simulink model "two_generators_loadFlow"  (R2014a)
settings: Solver=ode23tb  StartTime=0.0  StopTime=10  MaxStep=0.2  RelTol=1e-4
PreLoadFcn:
  | % -- Recommended Settings --
  | %
  | %  Simulink:
  | %      Solver: Ode23tb
  | %      Relative tolerance = 1e-4
  | %      Max step size = 0.2
  | %
  | %  Powergui:
  |          Ts = 0; % (continuous electrical model)
  | %
  | %
  | % ----------------------------------
undefined symbols (not defined in the file): D1, Delta
libraries: powerlib x6
settings Model: Creator=scastro  LastModifiedBy=cosorio
settings DebuggingCC: UnderspecifiedInitializationDetection=Classic  MultiTaskDSMMsg=warning  MultiTaskCondExecSysMsg=none  UnconnectedInputMsg=none  UnconnectedOutputMsg=none  UnconnectedLineMsg=none
settings RTWCC: IncludeERTFirstTime=on

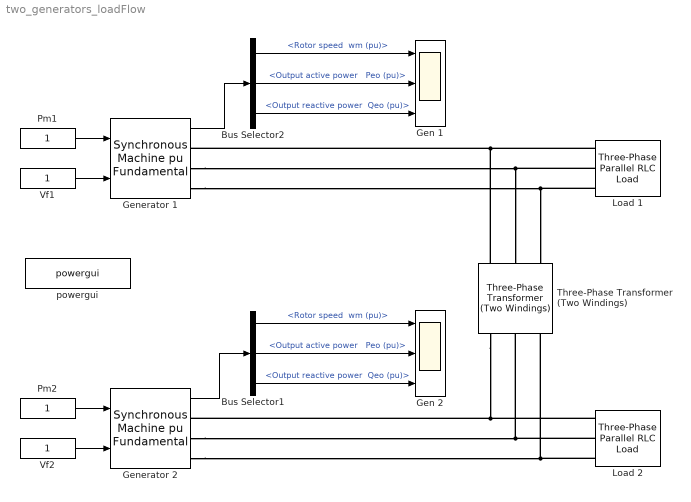
== system two_generators_loadFlow ==
  Bus Selector1 : BusSelector  OutputSignals="Mechanical.Rotor speed  wm (pu),Output active power   Peo (pu),Output reactive power  Qeo (pu)"
  Bus Selector2 : BusSelector  OutputSignals="Mechanical.Rotor speed  wm (pu),Output active power   Peo (pu),Output reactive power  Qeo (pu)"
  Gen 1 : Scope  NumInputPorts=3
      settings: YMin=0~0~0  YMax=2~2~2
  Gen 2 : Scope  NumInputPorts=3
      settings: YMin=0~0~0  YMax=2~2~2  SaveName=ScopeData2
  Generator 1 : powerlib/Machines/Synchronous Machine pu Fundamental  PresetModel=No  MechanicalLoad=Mechanical power Pm  ShowDetailedParameters=on  RotorType=Salient-pole  Units=per unit fundamental parameters  MeasurementBus=off  NominalParameters="[ 50e6  1200   60]"  Stator="[ 2.85E-03  0.114  1.19  0.36 ]"  Field="[ 5.79E-04  0.114]"  Dampers2=[0.0652, 0.5134, 0.0287, 0.2553, 7.765e-3, 0.9167 ]  Dampers1="[ 1.17E-02  0.182  1.97E-02  0.384 ]"  Mechanical=[ 4 0 4]  PolePairs=4  InitialConditions="[ 0  0  0  0  0  0  0  0  1 ]"  SetSaturation=off  Saturation=[0.6404,0.7127,0.8441,0.9214,0.9956,1.082,1.19,1.316,1.457;0.7,0.7698,0.8872,0.9466,0.9969,1.046,1.1,1.151,1.201]  LoadFlowParameters=[4 35000000 1200 0 15000000]  TsPowergui=0  TsBlock=-1  IterativeModel=Trapezoidal non iterative  BusType=swing  Pref=0  Qref=0  Qmin=-inf  Qmax=inf  PLF=0  QLF=0
      settings: AttributesFormatString=%<NominalParameters>
  Generator 2 : powerlib/Machines/Synchronous Machine pu Fundamental  PresetModel=No  MechanicalLoad=Mechanical power Pm  ShowDetailedParameters=on  RotorType=Salient-pole  Units=per unit fundamental parameters  MeasurementBus=off  NominalParameters="[ 50e6  2400   60]"  Stator="[ 2.85E-03  0.114  1.19  0.36 ]"  Field="[ 5.79E-04  0.114]"  Dampers2=[0.0652, 0.5134, 0.0287, 0.2553, 7.765e-3, 0.9167 ]  Dampers1="[ 1.17E-02  0.182  1.97E-02  0.384 ]"  Mechanical=[ 4 0 4]  PolePairs=4  InitialConditions="[ 0  0  0  0  0  0  0  0  1 ]"  SetSaturation=off  Saturation=[0.6404,0.7127,0.8441,0.9214,0.9956,1.082,1.19,1.316,1.457;0.7,0.7698,0.8872,0.9466,0.9969,1.046,1.1,1.151,1.201]  LoadFlowParameters=[2 40000000 1200 0 0]  TsPowergui=0  TsBlock=-1  IterativeModel=Trapezoidal non iterative  BusType=swing  Pref=0  Qref=0  Qmin=-inf  Qmax=inf  PLF=0  QLF=0
      settings: AttributesFormatString=%<NominalParameters>
  Load 1 : powerlib/Elements/Three-Phase Parallel RLC Load  LConnTagsString=A|B|C  Configuration=Y (grounded)  NominalVoltage=1200  NominalFrequency=60  ActivePower=40e6  InductivePower=0  CapacitivePower=0  Measurements=None  LoadType=constant Z
      settings: AttributesFormatString=|
      | P = %<ActivePower> W
      | Q = %<InductivePower> var
  Load 2 : powerlib/Elements/Three-Phase Parallel RLC Load  LConnTagsString=A|B|C  Configuration=Y (grounded)  NominalVoltage=2400  NominalFrequency=60  ActivePower=30e6  InductivePower=25e6  CapacitivePower=0  Measurements=None  LoadType=constant Z
      settings: AttributesFormatString=|
      | P = %<ActivePower> W
      | Q = %<InductivePower> var
  Pm1 : Constant
  Pm2 : Constant
  Three-Phase Transformer (Two Windings) : powerlib/Elements/Three-Phase Transformer (Two Windings)  Winding1Connection=Yg  UNITS=pu  NominalPower=[ 50e6 , 60 ]  Winding1=[ 2400 , 0.002 , 0.08 ]  Winding2Connection=Delta (D1)  Winding2=[ 1200 , 0.002 , 0.08 ]  SetSaturation=off  Rm=500  Lm=500  Saturation=[ 0,0 ; 0.0024,1.2 ; 1.0,1.52 ]  Hysteresis=off  DataFile='hysteresis'  SetInitialFlux=off  InitialFluxes=[ 0.8 , -0.8 , 0.7 ]  Measurements=None  MoreParameters=off  BreakLoop=off  DataType=off  TransfoNumber=1
  Vf1 : Constant
  Vf2 : Constant
  powergui : powerlib/powergui  Priority=1  SimulationMode=Continuous  SolverType=Tustin  SampleTime=1e-4  frequency=60  SPID=off  DisableSnubberDevices=off  DisableRonSwitches=off  DisableVfSwitches=off  SwTol=0  Interpol=off  DisplayEquations=off  Ts=0  methode=off  frequencyindice=60  Pbase=100e6  ErrMax=0.0001  Iterations=50  UnitsV=kV  UnitsW=MW  FunctionMessages=off  echomessages=off  HookPort=off  EnableUseOfTLC=off  x0status=blocks  RestoreLinks=warning  ResistiveCurrentMeasurement=off  Frange=[0:2:500]  Ylog=off  Xlog=on  ShowGrid=off  save=off  variable=ZData  structure=0  ZoomFFT=off  StartTime=0.0  cycles=1  DisplayStyle=1  fundamental=60  FreqAxis=off  MaxFrequency=1000  frequencyindicesteady=1  RmsSteady=1  display=off
  wires:
  Vf1/1 -> Generator 1/2
  Vf2/1 -> Generator 2/2
  Generator 2/1 -> Bus Selector1/1
  Bus Selector1/1 -> Gen 2/1  "<Rotor speed  wm (pu)>"
  Pm1/1 -> Generator 1/1
  Pm2/1 -> Generator 2/1
  Bus Selector1/2 -> Gen 2/2  "<Output active power   Peo (pu)>"
  Bus Selector1/3 -> Gen 2/3  "<Output reactive power  Qeo (pu)>"
  Generator 1/1 -> Bus Selector2/1
  Bus Selector2/1 -> Gen 1/1  "<Rotor speed  wm (pu)>"
  Bus Selector2/2 -> Gen 1/2  "<Output active power   Peo (pu)>"
  Bus Selector2/3 -> Gen 1/3  "<Output reactive power  Qeo (pu)>"
  connections:
  Three-Phase Transformer (Two Windings)/LConn1 -- Load 2/LConn1 -- Generator 2/RConn1
  Generator 1/RConn3 -- Three-Phase Transformer (Two Windings)/RConn3 -- Load 1/LConn3
  Generator 1/RConn2 -- Three-Phase Transformer (Two Windings)/RConn2 -- Load 1/LConn2
  Three-Phase Transformer (Two Windings)/RConn1 -- Load 1/LConn1 -- Generator 1/RConn1
  Generator 2/RConn2 -- Three-Phase Transformer (Two Windings)/LConn2 -- Load 2/LConn2
  Generator 2/RConn3 -- Three-Phase Transformer (Two Windings)/LConn3 -- Load 2/LConn3
